simulink model "Zbiorniki"  (Simulink 7.1)
settings: Solver=ode5  SolverMode=SingleTasking  StartTime=0.0  StopTime=999  FixedStep=T0  RelTol=1e-3  AbsTol=1e-6
values from neighbouring files (symbols this model uses):
  p1 = [15.5687861563 -0.119515470071]    [dane14listopad.mat]    (also in pomiary.m = polyfit(czujnik1,poziom1,1); pomiary11listopad.mat = [15.6445436161 -0.22526791704]; pomiary12listopad.mat = [15.6445436161 -0.22526791704])
  p2 = [15.4096010632 -0.0188344066907]    [dane14listopad.mat]    (also in pomiary.m = polyfit(czujnik2,poziom2,1); pomiary11listopad.mat = [15.42121958 -0.0351721095277]; pomiary12listopad.mat = [15.42121958 -0.0351721095277])
  p3 = [13.5370169173 -4.72805006493]    [dane14listopad.mat]    (also in pomiary.m = polyfit(czujnik3,poziom3,1); pomiary11listopad.mat = [24.705887162 -24.4919689549]; pomiary12listopad.mat = [24.705887162 -24.4919689549])
  T0 = 0.01    [dane14listopad.mat]    (also in daneZawory.mat; daneZawory_cz2.mat; pomiary11listopad.mat; pomiary12listopad.mat)
undefined symbols (not defined in the file or in its folder): mex_baseaddress
libraries: simulink x4
settings Model: Creator=jims  LastModifiedBy=lab  SimulationMode=external  ExtModeTrigDuration=300000
settings DataIOCC: ExternalInput=[]  InitialState=[]  LimitDataPoints=off  MaxDataPoints=5000  SaveOutput=off  SaveTime=off  SignalLoggingName=sigsOut
settings OptimizationCC: BooleanDataType=off
settings DebuggingCC: SaveWithParameterizedLinksMsg=none  SignalResolutionControl=TryResolveAllWithWarning  SolverPrmCheckMsg=none  MultiTaskDSMMsg=warning  MultiTaskCondExecSysMsg=none  IntegerOverflowMsg=none  StrictBusMsg=None
settings HardwareCC: TargetEndianess=LittleEndian  TargetHWDeviceType=MATLAB Host  ProdEqTarget=off
settings RTWCC: SystemTargetFile=rtwin.tlc  TemplateMakefile=rtwin.tmf  Description=Real-Time Windows Target  ProcessScript=rtwin_make_rtw_hook  IncludeERTFirstTime=on
settings RTWinTargetCC: TargetFunctionLibrary=ANSI_C  ModelReferenceCompliant=off  CompOptLevelCompliant=off  PortableWordSizes=off  CCOptimize=on

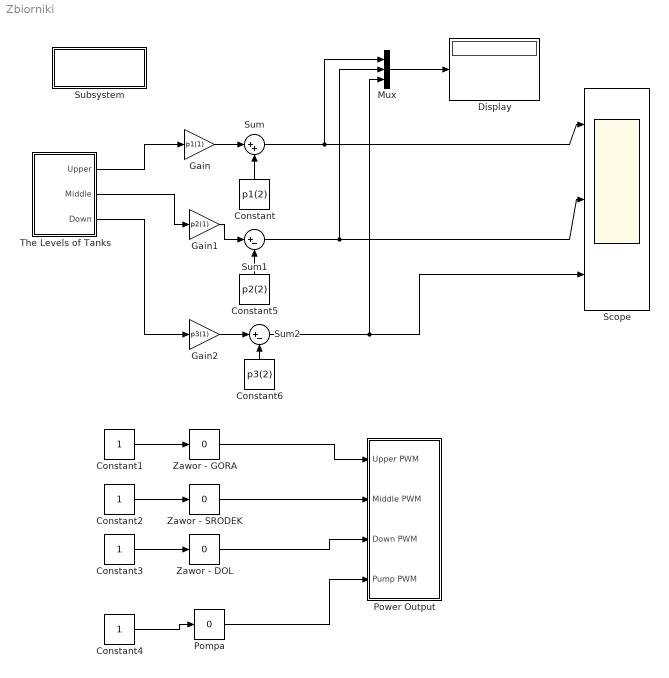
== system Zbiorniki ==
  Constant : Constant  Orientation=up  Value=p1(2)  OutDataType=sfix(16)  OutScaling=2^0
  Constant{1..4} (4 alike) : Constant  OutDataType=sfix(16)  OutScaling=2^0
  Constant5 : Constant  Orientation=up  Value=p2(2)  OutDataType=sfix(16)  OutScaling=2^0
  Constant6 : Constant  Orientation=up  Value=p3(2)  OutDataType=sfix(16)  OutScaling=2^0
  Display : Display
  Gain : Gain  Gain=p1(1)  ParameterDataType=sfix(16)  ParameterScaling=2^0  OutDataType=sfix(16)  OutScaling=2^0
  Gain1 : Gain  Gain=p2(1)  ParameterDataType=sfix(16)  ParameterScaling=2^0  OutDataType=sfix(16)  OutScaling=2^0
  Gain2 : Gain  Gain=p3(1)  ParameterDataType=sfix(16)  ParameterScaling=2^0  OutDataType=sfix(16)  OutScaling=2^0
  Mux : Mux  Inputs=3
  Pompa : simulink/Math Operations/Slider Gain  SystemSampleTime=-1  low=0  gain=0  high=1
  Power Output : Subsystem
  Scope : Scope  NumInputPorts=3
      settings: TimeRange=10  YMin=0.48~1.38778e-017~1.387  YMax=0.72~0.25~1.403  SaveName=Lev  MaxDataPoints=20000
  Subsystem : Subsystem
      settings: OpenFcn=T0=0.01
      mask Display: disp('Wczytaj T0')
  Sum : Sum  Inputs=|++  OutDataType=sfix(16)  OutScaling=2^0
  Sum1 : Sum  Inputs=|+-  OutDataType=sfix(16)  OutScaling=2^0
  Sum2 : Sum  Inputs=|+-  OutDataType=sfix(16)  OutScaling=2^0
  The Levels of Tanks : Subsystem
  Zawor - DOL : simulink/Math Operations/Slider Gain  SystemSampleTime=-1  low=0  gain=0  high=1
  Zawor - GORA : simulink/Math Operations/Slider Gain  SystemSampleTime=-1  low=0  gain=0  high=1
  Zawor - SRODEK : simulink/Math Operations/Slider Gain  SystemSampleTime=-1  low=0  gain=0  high=1
  wires:
  Mux/1 -> Display/1
  Constant2/1 -> Zawor - SRODEK/1
  Constant3/1 -> Zawor - DOL/1
  Zawor - SRODEK/1 -> Power Output/2(Middle PWM)
  Pompa/1 -> Power Output/4(Pump PWM)
  Constant1/1 -> Zawor - GORA/1
  Zawor - DOL/1 -> Power Output/3(Down PWM)
  Zawor - GORA/1 -> Power Output/1(Upper PWM)
  Constant4/1 -> Pompa/1
  The Levels of Tanks/3(Down) -> Gain2/1
  Constant5/1 -> Sum1/2
  The Levels of Tanks/1(Upper) -> Gain/1
  Sum/1 -> Scope/1, Mux/1
  Constant/1 -> Sum/2
  Gain/1 -> Sum/1
  Sum1/1 -> Scope/2, Mux/2
  The Levels of Tanks/2(Middle) -> Gain1/1
  Gain1/1 -> Sum1/1
  Sum2/1 -> Scope/3, Mux/3
  Constant6/1 -> Sum2/2
  Gain2/1 -> Sum2/1

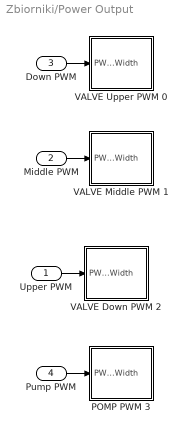
== system Zbiorniki/Power Output ==
  Upper PWM : Inport  OutDataType=sfix(16)  OutScaling=2^0
  Middle PWM : Inport  Port=2  OutDataType=sfix(16)  OutScaling=2^0
  Down PWM : Inport  Port=3  OutDataType=sfix(16)  OutScaling=2^0
  Pump PWM : Inport  Port=4  OutDataType=sfix(16)  OutScaling=2^0
  POMP PWM 3 : Subsystem  mask(PWM Module){BaseAddress=mex_baseaddress(-1,-1), ChanIdx=3, ChanMode=12 Bit, ChanPresc=30, SetOutputsFlag=on, SetOutputsValue=0, T0=T0}
      mask prompts: BaseAddress "IO Base Address:"; ChanIdx "Channel:"; ChanMode "Channel Mode:"; ChanPresc "Channel Prescaler:"; SetOutputsFlag "Set Outputs At Termination"; SetOutputsValue "Termination Outputs:"; T0 "Sample Time (sec):"
      mask help: RT-DAC PCI Device Driver
      mask Help: Set up each field for your specific hardware configuration.
      mask StyleString: edit,popup(0|1|2|3),popup(8 Bit|12 Bit),edit,checkbox,edit,edit
      mask Display: plot(0,0,100,100,[90,80,80,11,11],[90,90,20,20,80],[11,80],[80,80],[80,80],[20,14],[80,85,85,80],[45,45,66,66],[45,45,74,74],[20,13,13,20],[15,27,27,15,15],[75,75,26,26,75],[33,48,48,33,33],[75,75,55,55,75],[55,55,71,71,55],[55,75,75,55,55],[33,41,41,33,33],[50,50,27,27,50],[48,56,56,48,48],[50,50,27,27,50],[62,70,70,62,62],[50,50,27,27,50])
  VALVE Down PWM 2 : Subsystem  mask(PWM Module){BaseAddress=mex_baseaddress(-1,-1), ChanIdx=2, ChanMode=12 Bit, ChanPresc=30, SetOutputsFlag=on, SetOutputsValue=0, T0=T0}
      mask prompts: BaseAddress "IO Base Address:"; ChanIdx "Channel:"; ChanMode "Channel Mode:"; ChanPresc "Channel Prescaler:"; SetOutputsFlag "Set Outputs At Termination"; SetOutputsValue "Termination Outputs:"; T0 "Sample Time (sec):"
      mask help: RT-DAC PCI Device Driver
      mask Help: Set up each field for your specific hardware configuration.
      mask StyleString: edit,popup(0|1|2|3),popup(8 Bit|12 Bit),edit,checkbox,edit,edit
      mask Display: plot(0,0,100,100,[90,80,80,11,11],[90,90,20,20,80],[11,80],[80,80],[80,80],[20,14],[80,85,85,80],[45,45,66,66],[45,45,74,74],[20,13,13,20],[15,27,27,15,15],[75,75,26,26,75],[33,48,48,33,33],[75,75,55,55,75],[55,55,71,71,55],[55,75,75,55,55],[33,41,41,33,33],[50,50,27,27,50],[48,56,56,48,48],[50,50,27,27,50],[62,70,70,62,62],[50,50,27,27,50])
  VALVE Middle PWM 1 : Subsystem  mask(PWM Module){BaseAddress=mex_baseaddress(-1,-1), ChanIdx=1, ChanMode=12 Bit, ChanPresc=30, SetOutputsFlag=on, SetOutputsValue=0, T0=T0}
      mask prompts: BaseAddress "IO Base Address:"; ChanIdx "Channel:"; ChanMode "Channel Mode:"; ChanPresc "Channel Prescaler:"; SetOutputsFlag "Set Outputs At Termination"; SetOutputsValue "Termination Outputs:"; T0 "Sample Time (sec):"
      mask help: RT-DAC PCI Device Driver
      mask Help: Set up each field for your specific hardware configuration.
      mask StyleString: edit,popup(0|1|2|3),popup(8 Bit|12 Bit),edit,checkbox,edit,edit
      mask Display: plot(0,0,100,100,[90,80,80,11,11],[90,90,20,20,80],[11,80],[80,80],[80,80],[20,14],[80,85,85,80],[45,45,66,66],[45,45,74,74],[20,13,13,20],[15,27,27,15,15],[75,75,26,26,75],[33,48,48,33,33],[75,75,55,55,75],[55,55,71,71,55],[55,75,75,55,55],[33,41,41,33,33],[50,50,27,27,50],[48,56,56,48,48],[50,50,27,27,50],[62,70,70,62,62],[50,50,27,27,50])
  VALVE Upper PWM 0 : Subsystem  mask(PWM Module){BaseAddress=mex_baseaddress(-1,-1), ChanIdx=0, ChanMode=12 Bit, ChanPresc=30, SetOutputsFlag=on, SetOutputsValue=0, T0=T0}
      mask prompts: BaseAddress "IO Base Address:"; ChanIdx "Channel:"; ChanMode "Channel Mode:"; ChanPresc "Channel Prescaler:"; SetOutputsFlag "Set Outputs At Termination"; SetOutputsValue "Termination Outputs:"; T0 "Sample Time (sec):"
      mask help: RT-DAC PCI Device Driver
      mask Help: Set up each field for your specific hardware configuration.
      mask StyleString: edit,popup(0|1|2|3),popup(8 Bit|12 Bit),edit,checkbox,edit,edit
      mask Display: plot(0,0,100,100,[90,80,80,11,11],[90,90,20,20,80],[11,80],[80,80],[80,80],[20,14],[80,85,85,80],[45,45,66,66],[45,45,74,74],[20,13,13,20],[15,27,27,15,15],[75,75,26,26,75],[33,48,48,33,33],[75,75,55,55,75],[55,55,71,71,55],[55,75,75,55,55],[33,41,41,33,33],[50,50,27,27,50],[48,56,56,48,48],[50,50,27,27,50],[62,70,70,62,62],[50,50,27,27,50])
  wires:
  Down PWM/1 -> VALVE Upper PWM 0/1(PWM Width)
  Middle PWM/1 -> VALVE Middle PWM 1/1(PWM Width)
  Upper PWM/1 -> VALVE Down PWM 2/1(PWM Width)
  Pump PWM/1 -> POMP PWM 3/1(PWM Width)

== system Zbiorniki/Subsystem ==

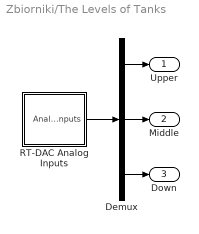
== system Zbiorniki/The Levels of Tanks ==
  Demux : Demux  Outputs=3
  RT-DAC Analog Inputs : Subsystem  mask( Analog Input Module){BaseAddress=mex_baseaddress(-1,-1), Chan=[0 1 2], Gain=[1 1 1], T0=0.05}
      mask prompts: BaseAddress "Base Address:"; Chan "Channel:"; T0 "Sample Time (sec):"
      mask help: RT-DAC PCI Device Driver
      mask Help: Set up each field for your specific hardware configuration.
      mask Display: plot(0,0,100,100,[90,80,80,11,11],[90,90,20,20,80],[11,80],[80,80],[80,80],[20,14],[80,85,85,80],[45,45,66,66],[45,45,74,74],[20,13,13,20],[15,27,27,15,15],[75,75,26,26,75],[33,48,48,33,33],[75,75,55,55,75],[55,55,71,71,55],[55,75,75,55,55],[33,41,41,33,33],[50,50,27,27,50],[48,56,56,48,48],[50,50,27,27,50],[62,70,70,62,62],[50,50,27,27,50])
  Upper : Outport
  Middle : Outport  Port=2
  Down : Outport  Port=3
  wires:
  RT-DAC Analog Inputs/1(Analog Inputs) -> Demux/1
  Demux/1 -> Upper/1
  Demux/2 -> Middle/1
  Demux/3 -> Down/1

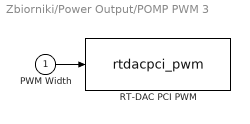
== system Zbiorniki/Power Output/POMP PWM 3 ==
  PWM Width : Inport  OutDataType=sfix(16)  OutScaling=2^0
  "RT-DAC PCI PWM " : S-Function  FunctionName=rtdacpci_pwm  Parameters=BaseAddress, ChanIdx, ChanMode, ChanPresc, SetOutputsFlag, SetOutputsValue, T0  EnableBusSupport=off
  wires:
  PWM Width/1 -> "RT-DAC PCI PWM "/1

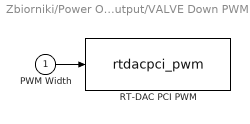
== system Zbiorniki/Power Output/VALVE Down PWM 2 ==
  PWM Width : Inport  OutDataType=sfix(16)  OutScaling=2^0
  "RT-DAC PCI PWM " : S-Function  FunctionName=rtdacpci_pwm  Parameters=BaseAddress, ChanIdx, ChanMode, ChanPresc, SetOutputsFlag, SetOutputsValue, T0  EnableBusSupport=off
  wires:
  PWM Width/1 -> "RT-DAC PCI PWM "/1

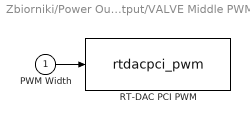
== system Zbiorniki/Power Output/VALVE Middle PWM 1 ==
  PWM Width : Inport  OutDataType=sfix(16)  OutScaling=2^0
  "RT-DAC PCI PWM " : S-Function  FunctionName=rtdacpci_pwm  Parameters=BaseAddress, ChanIdx, ChanMode, ChanPresc, SetOutputsFlag, SetOutputsValue, T0  EnableBusSupport=off
  wires:
  PWM Width/1 -> "RT-DAC PCI PWM "/1

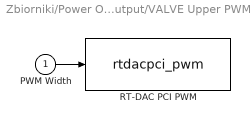
== system Zbiorniki/Power Output/VALVE Upper PWM 0 ==
  PWM Width : Inport  OutDataType=sfix(16)  OutScaling=2^0
  "RT-DAC PCI PWM " : S-Function  FunctionName=rtdacpci_pwm  Parameters=BaseAddress, ChanIdx, ChanMode, ChanPresc, SetOutputsFlag, SetOutputsValue, T0  EnableBusSupport=off
  wires:
  PWM Width/1 -> "RT-DAC PCI PWM "/1

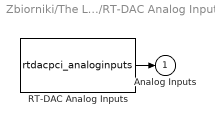
== system Zbiorniki/The Levels of Tanks/RT-DAC Analog Inputs ==
  RT-DAC Analog Inputs : S-Function  FunctionName=rtdacpci_analoginputs  Parameters=BaseAddress, Chan, Gain, T0  EnableBusSupport=off
  Analog Inputs : Outport
  wires:
  RT-DAC Analog Inputs/1 -> Analog Inputs/1
